simulink model "mcdc_test_tmp"  (Simulink 8.8)
settings: Solver=FixedStepDiscrete  StartTime=0.0  StopTime=10.0  RelTol=1e-3  EnableMultiTasking=on
settings Model: Creator=arnaud  LastModifiedBy=hbourbou
settings DataIOCC: SaveFormat=Structure
settings OptimizationCC: ExpressionDepthLimit=2147483647
settings DebuggingCC: SolverPrmCheckMsg=warning
settings ConfigComp: CovSFcnEnable=off

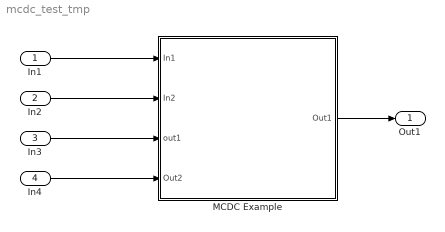
== system mcdc_test_tmp ==
  In1 : Inport  OutDataTypeStr=int32
  In2 : Inport  Port=2  OutDataTypeStr=int32
  In3 : Inport  Port=3  OutDataTypeStr=int32
  In4 : Inport  Port=4  OutDataTypeStr=int32
  MCDC Example : Subsystem  TreatAsAtomicUnit=on
      settings: MinAlgLoopOccurrences=on
  Out1 : Outport
  wires:
  MCDC Example/1(Out1) -> Out1/1
  In1/1 -> MCDC Example/1(In1)
  In2/1 -> MCDC Example/2(In2)
  In3/1 -> MCDC Example/3(out1)
  In4/1 -> MCDC Example/4(Out2)

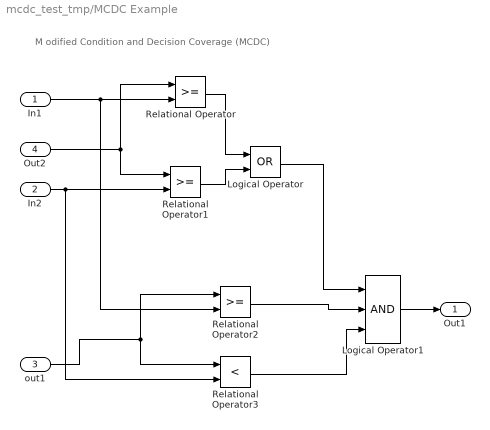
== system mcdc_test_tmp/MCDC Example ==
  note: M odified Condition and Decision Coverage (MCDC)
  In1 : Inport
  In2 : Inport  Port=2
  out1 : Inport  Port=3
  Out2 : Inport  Port=4
  Logical Operator : Logic  Operator=OR  AllPortsSameDT=off  OutDataTypeStr=boolean
  Logical Operator1 : Logic  Inputs=3  AllPortsSameDT=off  OutDataTypeStr=boolean
  Relational Operator : RelationalOperator  OutDataTypeStr=boolean  RndMeth=Nearest
  Relational Operator1 : RelationalOperator  OutDataTypeStr=boolean  RndMeth=Nearest
  Relational Operator2 : RelationalOperator  OutDataTypeStr=boolean  RndMeth=Nearest
  Relational Operator3 : RelationalOperator  Operator=<  OutDataTypeStr=boolean  RndMeth=Nearest
  Out1 : Outport
  wires:
  Relational Operator/1 -> Logical Operator/1
  Relational Operator1/1 -> Logical Operator/2
  Logical Operator/1 -> Logical Operator1/1
  Out2/1 -> Relational Operator/1, Relational Operator1/1
  Logical Operator1/1 -> Out1/1
  Relational Operator2/1 -> Logical Operator1/2
  Relational Operator3/1 -> Logical Operator1/3
  out1/1 -> Relational Operator2/1, Relational Operator3/1
  In2/1 -> Relational Operator3/2, Relational Operator1/2
  In1/1 -> Relational Operator2/2, Relational Operator/2
